simulink subsystem "MFTiresMultibodySSC"  (R2024b)
settings: Solver=VariableStepAuto  StartTime=0.0  StopTime=10.0  RelTol=1e-3
undefined symbols (not defined in the file): AxlFL, AxlFR, AxlRL, AxlRR, PlntVehMultiBody, WheelFL, WheelFR, WheelRL, WheelRR, X, Y, Z
libraries: sm_lib x68, nesl_utility x52, fl_lib x8
(part 3 of 3)

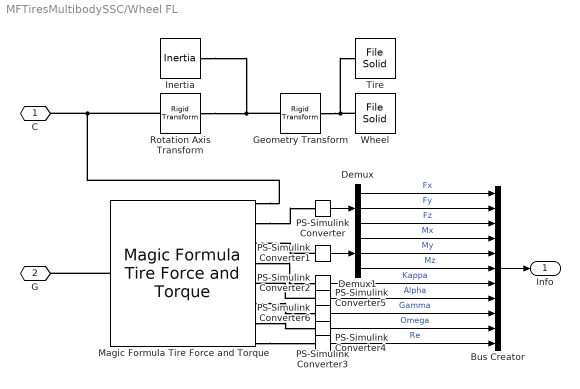
== system MFTiresMultibodySSC/Wheel FL ==
  Bus Creator : BusCreator  Inputs=11
  Demux : Demux  Outputs=3
  Demux1 : Demux  Outputs=3
  Geometry Transform : sm_lib/Frames and Transforms/Rigid Transform  RotationMethod=StandardAxis  FollAlignAxisA=+X  BaseAlignAxisA=+Y  FollAlignAxisB=+Y  BaseAlignAxisB=+Z  RotationStandardAxis=+X  RotationAngle=sideSign*180-90  RotationAngleUnits=deg  RotationArbitraryAxis=[0 0 1]  RotationSequenceAxes=FollowerAxes  RotationSequence=XYX  RotationSequenceAngles=[0 0 0]  RotationSequenceAnglesUnits=deg  RotationMatrix=[1 0 0; 0 1 0; 0 0 1]  Quaternion=[1 0 0 0]  TranslationMethod=StandardAxis  TranslationCartesianOffset=[0 0 0]  TranslationCartesianOffsetUnits=m  TranslationStandardAxis=+Y  TranslationStandardOffset=(1-2*sideSign)*0.125  TranslationStandardOffsetUnits=m  TranslationROffset=0  TranslationROffsetUnits=m  TranslationThetaOffset=0  TranslationThetaOffsetUnits=deg  TranslationZOffset=0  TranslationZOffsetUnits=m
  Inertia : sm_lib/Body Elements/Inertia  InertiaType=Custom  Mass=wheelAssm_mass  MassUnits=kg  CenterOfMass=[0 0 0]  CenterOfMassUnits=m  MomentsOfInertia=wheelAssm_I  MomentsOfInertiaUnits=kg*m^2  ProductsOfInertia=[0 0 0]  ProductsOfInertiaUnits=kg*m^2  GraphicType=None  MarkerShape=Inertia  MarkerSize=20  GraphicVisPropType=SimpleVisualProperties  GraphicDiffuseColor=[0.5 0.5 0.5]  GraphicOpacity=1.0  GraphicSpecularColor=[0.5 0.5 0.5 1.0]  GraphicAmbientColor=[0.15 0.15 0.15 1.0]  GraphicEmissiveColor=[0.0 0.0 0.0 1.0]  GraphicShininess=75
  Magic Formula Tire Force and Torque : sm_lib/Forces and Torques/Magic Formula Tire Force and Torque  TireSide=Left  TireParameters=tire_param  SlipMode=Combined  ContactFrameMethod=ClosestPoint  ScalingCoefficientLMUXMode=FromTireParameters  ScalingCoefficientLMUYMode=FromTireParameters  SenseContactSignal=off  TireWrenchFrame=ContactFrame  SenseTireForce=on  SenseTireTorque=on  SensePneumaticTrail=off  SenseLongitudinalSlip=on  SenseSaturatedLongitudinalSlip=off  SenseSlipAngle=on  SenseSaturatedSlipAngle=off  SenseTurnSlip=off  SenseRelativeLongitudinalVelocity=off  SenseRelativeLateralVelocity=off  SenseLongitudinalSlipVelocity=off  SenseLateralSlipVelocity=off  SenseYawVelocity=off  SenseCamberAngle=on  SenseSaturatedCamberAngle=off  SenseCamberVelocity=off  SenseSpinVelocity=on  SenseFreeRadius=off  SenseLoadedRadius=off  SenseEffectiveRollingRadius=on  SenseRadialDeflection=off  SenseLongitudinalFrictionCoefficient=off  SenseLateralFrictionCoefficient=off  SenseContactBaseRotation=off  SenseContactBaseTranslation=off  SenseContactFollowerRotation=off  SenseContactFollowerTranslation=off  NumericParameters=[0.1 0.1 0.1 0.1 0.1 1e-4 1e-4 1e-7 1e-7 1e-4 1e-4 0.1 1e-4 1e-4 1e-4 1e-4 1e-4 1e-4 1e-4 1e-4 1e-4]
  PS-Simulink Converter{,1..6} (7 alike) : nesl_utility/PS-Simulink Converter  PhysicalDomain=network_engine_domain  SubClassName=ps_output  LeftPortType=input  RightPortType=output  PseudoPeriodic=off  Frequencies=[]  VectorFormat=1-D array  Unit=inherit  AffineConversion=off
  Rotation Axis Transform : sm_lib/Frames and Transforms/Rigid Transform  RotationMethod=AlignedAxes  FollAlignAxisA=+X  BaseAlignAxisA=+X  FollAlignAxisB=+Z  BaseAlignAxisB=+Y  RotationStandardAxis=-X  RotationAngle=0  RotationAngleUnits=deg  RotationArbitraryAxis=[0 0 1]  RotationSequenceAxes=FollowerAxes  RotationSequence=XYX  RotationSequenceAngles=[0 0 0]  RotationSequenceAnglesUnits=deg  RotationMatrix=[1 0 0; 0 1 0; 0 0 1]  Quaternion=[1 0 0 0]  TranslationMethod=None  TranslationCartesianOffset=[0 0 0]  TranslationCartesianOffsetUnits=m  TranslationStandardAxis=+Z  TranslationStandardOffset=0  TranslationStandardOffsetUnits=m  TranslationROffset=0  TranslationROffsetUnits=m  TranslationThetaOffset=0  TranslationThetaOffsetUnits=deg  TranslationZOffset=0  TranslationZOffsetUnits=m
  Tire : sm_lib/Body Elements/File Solid  ExtGeomFileName=sm_car_heave_roll_tire.STL  UnitType=Custom  ExtGeomFileUnits=mm  StepReaderType=HEX  ExportConvexHullGeometry=off  InertiaType=Custom  BasedOnType=Density  Density=1000  DensityUnits=kg/m^3  Mass=0  MassUnits=kg  CenterOfMass=[0 0 0]  CenterOfMassUnits=m  MomentsOfInertia=[0 0 0]  MomentsOfInertiaUnits=kg*m^2  ProductsOfInertia=[0 0 0]  ProductsOfInertiaUnits=kg*m^2  GraphicType=FromGeometry  MarkerShape=Sphere  MarkerSize=10  GraphicVisPropType=SimpleVisualProperties  GraphicDiffuseColor=[0.5 0.5 0.5]  GraphicOpacity=1.0  GraphicSpecularColor=[0.5 0.5 0.5 1.0]  GraphicAmbientColor=[0.15 0.15 0.15 1.0]  GraphicEmissiveColor=[0.0 0.0 0.0 1.0]  GraphicShininess=75  DoExposeReferenceFrame=on  SerializedFrames=<Frames/>
  Wheel : sm_lib/Body Elements/File Solid  ExtGeomFileName=sm_car_heave_roll_wheel.STL  UnitType=Custom  ExtGeomFileUnits=mm  StepReaderType=HEX  ExportConvexHullGeometry=off  InertiaType=Custom  BasedOnType=Density  Density=1000  DensityUnits=kg/m^3  Mass=0  MassUnits=kg  CenterOfMass=[0 0 0]  CenterOfMassUnits=m  MomentsOfInertia=[0 0 0]  MomentsOfInertiaUnits=kg*m^2  ProductsOfInertia=[0 0 0]  ProductsOfInertiaUnits=kg*m^2  GraphicType=FromGeometry  MarkerShape=Sphere  MarkerSize=10  GraphicVisPropType=SimpleVisualProperties  GraphicDiffuseColor=[0.8 0.8 0.8]  GraphicOpacity=1.0  GraphicSpecularColor=[0.5 0.5 0.5 1.0]  GraphicAmbientColor=[0.15 0.15 0.15 1.0]  GraphicEmissiveColor=[0.0 0.0 0.0 1.0]  GraphicShininess=75  DoExposeReferenceFrame=on  SerializedFrames=<Frames/>
  C : PMIOPort  Side=Left
  G : PMIOPort  Port=2  Side=Right
  Info : Outport
  wires:
  PS-Simulink Converter5/1 -> Bus Creator/8  "Alpha"
  PS-Simulink Converter4/1 -> Bus Creator/11  "Re"
  PS-Simulink Converter3/1 -> Bus Creator/10  "Omega"
  PS-Simulink Converter2/1 -> Bus Creator/7  "Kappa"
  PS-Simulink Converter/1 -> Demux/1
  Demux/1 -> Bus Creator/1  "Fx"
  Demux/2 -> Bus Creator/2  "Fy"
  Demux/3 -> Bus Creator/3  "Fz"
  Demux1/3 -> Bus Creator/6  "Mz"
  Demux1/2 -> Bus Creator/5  "My"
  Demux1/1 -> Bus Creator/4  "Mx"
  PS-Simulink Converter1/1 -> Demux1/1
  Bus Creator/1 -> Info/1
  PS-Simulink Converter6/1 -> Bus Creator/9  "Gamma"
  connections:
  PS-Simulink Converter5/LConn1 -- Magic Formula Tire Force and Torque/RConn5
  Magic Formula Tire Force and Torque/RConn7 -- PS-Simulink Converter3/LConn1
  Magic Formula Tire Force and Torque/RConn8 -- PS-Simulink Converter4/LConn1
  Magic Formula Tire Force and Torque/RConn4 -- PS-Simulink Converter2/LConn1
  Wheel/RConn1 -- Geometry Transform/RConn1 -- Tire/RConn1
  Inertia/RConn1 -- Geometry Transform/LConn1 -- Rotation Axis Transform/LConn1
  Magic Formula Tire Force and Torque/LConn1 -- G/RConn1
  Magic Formula Tire Force and Torque/RConn2 -- PS-Simulink Converter/LConn1
  PS-Simulink Converter1/LConn1 -- Magic Formula Tire Force and Torque/RConn3
  Rotation Axis Transform/RConn1 -- Magic Formula Tire Force and Torque/RConn1 -- C/RConn1
  Magic Formula Tire Force and Torque/RConn6 -- PS-Simulink Converter6/LConn1

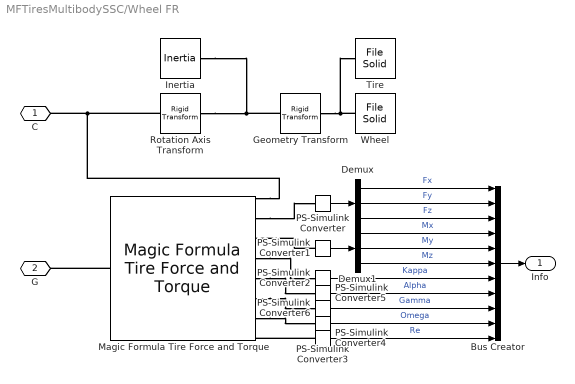
== system MFTiresMultibodySSC/Wheel FR ==
  Bus Creator : BusCreator  Inputs=11
  Demux : Demux  Outputs=3
  Demux1 : Demux  Outputs=3
  Geometry Transform : sm_lib/Frames and Transforms/Rigid Transform  RotationMethod=StandardAxis  FollAlignAxisA=+X  BaseAlignAxisA=+Y  FollAlignAxisB=+Y  BaseAlignAxisB=+Z  RotationStandardAxis=+X  RotationAngle=sideSign*180-90  RotationAngleUnits=deg  RotationArbitraryAxis=[0 0 1]  RotationSequenceAxes=FollowerAxes  RotationSequence=XYX  RotationSequenceAngles=[0 0 0]  RotationSequenceAnglesUnits=deg  RotationMatrix=[1 0 0; 0 1 0; 0 0 1]  Quaternion=[1 0 0 0]  TranslationMethod=StandardAxis  TranslationCartesianOffset=[0 0 0]  TranslationCartesianOffsetUnits=m  TranslationStandardAxis=+Y  TranslationStandardOffset=(1-2*sideSign)*0.125  TranslationStandardOffsetUnits=m  TranslationROffset=0  TranslationROffsetUnits=m  TranslationThetaOffset=0  TranslationThetaOffsetUnits=deg  TranslationZOffset=0  TranslationZOffsetUnits=m
  Inertia : sm_lib/Body Elements/Inertia  InertiaType=Custom  Mass=wheelAssm_mass  MassUnits=kg  CenterOfMass=[0 0 0]  CenterOfMassUnits=m  MomentsOfInertia=wheelAssm_I  MomentsOfInertiaUnits=kg*m^2  ProductsOfInertia=[0 0 0]  ProductsOfInertiaUnits=kg*m^2  GraphicType=None  MarkerShape=Inertia  MarkerSize=20  GraphicVisPropType=SimpleVisualProperties  GraphicDiffuseColor=[0.5 0.5 0.5]  GraphicOpacity=1.0  GraphicSpecularColor=[0.5 0.5 0.5 1.0]  GraphicAmbientColor=[0.15 0.15 0.15 1.0]  GraphicEmissiveColor=[0.0 0.0 0.0 1.0]  GraphicShininess=75
  Magic Formula Tire Force and Torque : sm_lib/Forces and Torques/Magic Formula Tire Force and Torque  TireSide=Right  TireParameters=tire_param  SlipMode=Combined  ContactFrameMethod=ClosestPoint  ScalingCoefficientLMUXMode=FromTireParameters  ScalingCoefficientLMUYMode=FromTireParameters  SenseContactSignal=off  TireWrenchFrame=ContactFrame  SenseTireForce=on  SenseTireTorque=on  SensePneumaticTrail=off  SenseLongitudinalSlip=on  SenseSaturatedLongitudinalSlip=off  SenseSlipAngle=on  SenseSaturatedSlipAngle=off  SenseTurnSlip=off  SenseRelativeLongitudinalVelocity=off  SenseRelativeLateralVelocity=off  SenseLongitudinalSlipVelocity=off  SenseLateralSlipVelocity=off  SenseYawVelocity=off  SenseCamberAngle=on  SenseSaturatedCamberAngle=off  SenseCamberVelocity=off  SenseSpinVelocity=on  SenseFreeRadius=off  SenseLoadedRadius=off  SenseEffectiveRollingRadius=on  SenseRadialDeflection=off  SenseLongitudinalFrictionCoefficient=off  SenseLateralFrictionCoefficient=off  SenseContactBaseRotation=off  SenseContactBaseTranslation=off  SenseContactFollowerRotation=off  SenseContactFollowerTranslation=off  NumericParameters=[0.1 0.1 0.1 0.1 0.1 1e-4 1e-4 1e-7 1e-7 1e-4 1e-4 0.1 1e-4 1e-4 1e-4 1e-4 1e-4 1e-4 1e-4 1e-4 1e-4]
  PS-Simulink Converter{,1..6} (7 alike) : nesl_utility/PS-Simulink Converter  PhysicalDomain=network_engine_domain  SubClassName=ps_output  LeftPortType=input  RightPortType=output  PseudoPeriodic=off  Frequencies=[]  VectorFormat=1-D array  Unit=inherit  AffineConversion=off
  Rotation Axis Transform : sm_lib/Frames and Transforms/Rigid Transform  RotationMethod=AlignedAxes  FollAlignAxisA=+X  BaseAlignAxisA=+X  FollAlignAxisB=+Z  BaseAlignAxisB=+Y  RotationStandardAxis=-X  RotationAngle=0  RotationAngleUnits=deg  RotationArbitraryAxis=[0 0 1]  RotationSequenceAxes=FollowerAxes  RotationSequence=XYX  RotationSequenceAngles=[0 0 0]  RotationSequenceAnglesUnits=deg  RotationMatrix=[1 0 0; 0 1 0; 0 0 1]  Quaternion=[1 0 0 0]  TranslationMethod=None  TranslationCartesianOffset=[0 0 0]  TranslationCartesianOffsetUnits=m  TranslationStandardAxis=+Z  TranslationStandardOffset=0  TranslationStandardOffsetUnits=m  TranslationROffset=0  TranslationROffsetUnits=m  TranslationThetaOffset=0  TranslationThetaOffsetUnits=deg  TranslationZOffset=0  TranslationZOffsetUnits=m
  Tire : sm_lib/Body Elements/File Solid  ExtGeomFileName=sm_car_heave_roll_tire.STL  UnitType=Custom  ExtGeomFileUnits=mm  StepReaderType=HEX  ExportConvexHullGeometry=off  InertiaType=Custom  BasedOnType=Density  Density=1000  DensityUnits=kg/m^3  Mass=0  MassUnits=kg  CenterOfMass=[0 0 0]  CenterOfMassUnits=m  MomentsOfInertia=[0 0 0]  MomentsOfInertiaUnits=kg*m^2  ProductsOfInertia=[0 0 0]  ProductsOfInertiaUnits=kg*m^2  GraphicType=FromGeometry  MarkerShape=Sphere  MarkerSize=10  GraphicVisPropType=SimpleVisualProperties  GraphicDiffuseColor=[0.5 0.5 0.5]  GraphicOpacity=1.0  GraphicSpecularColor=[0.5 0.5 0.5 1.0]  GraphicAmbientColor=[0.15 0.15 0.15 1.0]  GraphicEmissiveColor=[0.0 0.0 0.0 1.0]  GraphicShininess=75  DoExposeReferenceFrame=on  SerializedFrames=<Frames/>
  Wheel : sm_lib/Body Elements/File Solid  ExtGeomFileName=sm_car_heave_roll_wheel.STL  UnitType=Custom  ExtGeomFileUnits=mm  StepReaderType=HEX  ExportConvexHullGeometry=off  InertiaType=Custom  BasedOnType=Density  Density=1000  DensityUnits=kg/m^3  Mass=0  MassUnits=kg  CenterOfMass=[0 0 0]  CenterOfMassUnits=m  MomentsOfInertia=[0 0 0]  MomentsOfInertiaUnits=kg*m^2  ProductsOfInertia=[0 0 0]  ProductsOfInertiaUnits=kg*m^2  GraphicType=FromGeometry  MarkerShape=Sphere  MarkerSize=10  GraphicVisPropType=SimpleVisualProperties  GraphicDiffuseColor=[0.8 0.8 0.8]  GraphicOpacity=1.0  GraphicSpecularColor=[0.5 0.5 0.5 1.0]  GraphicAmbientColor=[0.15 0.15 0.15 1.0]  GraphicEmissiveColor=[0.0 0.0 0.0 1.0]  GraphicShininess=75  DoExposeReferenceFrame=on  SerializedFrames=<Frames/>
  C : PMIOPort  Side=Left
  G : PMIOPort  Port=2  Side=Right
  Info : Outport
  wires:
  PS-Simulink Converter5/1 -> Bus Creator/8  "Alpha"
  PS-Simulink Converter4/1 -> Bus Creator/11  "Re"
  PS-Simulink Converter3/1 -> Bus Creator/10  "Omega"
  PS-Simulink Converter2/1 -> Bus Creator/7  "Kappa"
  PS-Simulink Converter/1 -> Demux/1
  Demux/1 -> Bus Creator/1  "Fx"
  Demux/2 -> Bus Creator/2  "Fy"
  Demux/3 -> Bus Creator/3  "Fz"
  Demux1/3 -> Bus Creator/6  "Mz"
  Demux1/2 -> Bus Creator/5  "My"
  Demux1/1 -> Bus Creator/4  "Mx"
  PS-Simulink Converter1/1 -> Demux1/1
  Bus Creator/1 -> Info/1
  PS-Simulink Converter6/1 -> Bus Creator/9  "Gamma"
  connections:
  Magic Formula Tire Force and Torque/RConn5 -- PS-Simulink Converter5/LConn1
  PS-Simulink Converter4/LConn1 -- Magic Formula Tire Force and Torque/RConn8
  Magic Formula Tire Force and Torque/RConn7 -- PS-Simulink Converter3/LConn1
  Magic Formula Tire Force and Torque/RConn4 -- PS-Simulink Converter2/LConn1
  Wheel/RConn1 -- Geometry Transform/RConn1 -- Tire/RConn1
  Inertia/RConn1 -- Geometry Transform/LConn1 -- Rotation Axis Transform/LConn1
  Magic Formula Tire Force and Torque/LConn1 -- G/RConn1
  Magic Formula Tire Force and Torque/RConn2 -- PS-Simulink Converter/LConn1
  PS-Simulink Converter1/LConn1 -- Magic Formula Tire Force and Torque/RConn3
  Rotation Axis Transform/RConn1 -- Magic Formula Tire Force and Torque/RConn1 -- C/RConn1
  Magic Formula Tire Force and Torque/RConn6 -- PS-Simulink Converter6/LConn1

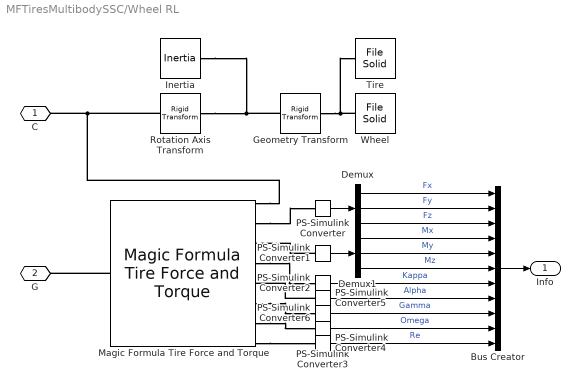
== system MFTiresMultibodySSC/Wheel RL ==
  Bus Creator : BusCreator  Inputs=11
  Demux : Demux  Outputs=3
  Demux1 : Demux  Outputs=3
  Geometry Transform : sm_lib/Frames and Transforms/Rigid Transform  RotationMethod=StandardAxis  FollAlignAxisA=+X  BaseAlignAxisA=+Y  FollAlignAxisB=+Y  BaseAlignAxisB=+Z  RotationStandardAxis=+X  RotationAngle=sideSign*180-90  RotationAngleUnits=deg  RotationArbitraryAxis=[0 0 1]  RotationSequenceAxes=FollowerAxes  RotationSequence=XYX  RotationSequenceAngles=[0 0 0]  RotationSequenceAnglesUnits=deg  RotationMatrix=[1 0 0; 0 1 0; 0 0 1]  Quaternion=[1 0 0 0]  TranslationMethod=StandardAxis  TranslationCartesianOffset=[0 0 0]  TranslationCartesianOffsetUnits=m  TranslationStandardAxis=+Y  TranslationStandardOffset=(1-2*sideSign)*0.125  TranslationStandardOffsetUnits=m  TranslationROffset=0  TranslationROffsetUnits=m  TranslationThetaOffset=0  TranslationThetaOffsetUnits=deg  TranslationZOffset=0  TranslationZOffsetUnits=m
  Inertia : sm_lib/Body Elements/Inertia  InertiaType=Custom  Mass=wheelAssm_mass  MassUnits=kg  CenterOfMass=[0 0 0]  CenterOfMassUnits=m  MomentsOfInertia=wheelAssm_I  MomentsOfInertiaUnits=kg*m^2  ProductsOfInertia=[0 0 0]  ProductsOfInertiaUnits=kg*m^2  GraphicType=None  MarkerShape=Inertia  MarkerSize=20  GraphicVisPropType=SimpleVisualProperties  GraphicDiffuseColor=[0.5 0.5 0.5]  GraphicOpacity=1.0  GraphicSpecularColor=[0.5 0.5 0.5 1.0]  GraphicAmbientColor=[0.15 0.15 0.15 1.0]  GraphicEmissiveColor=[0.0 0.0 0.0 1.0]  GraphicShininess=75
  Magic Formula Tire Force and Torque : sm_lib/Forces and Torques/Magic Formula Tire Force and Torque  TireSide=Left  TireParameters=tire_param  SlipMode=Combined  ContactFrameMethod=ClosestPoint  ScalingCoefficientLMUXMode=FromTireParameters  ScalingCoefficientLMUYMode=FromTireParameters  SenseContactSignal=off  TireWrenchFrame=ContactFrame  SenseTireForce=on  SenseTireTorque=on  SensePneumaticTrail=off  SenseLongitudinalSlip=on  SenseSaturatedLongitudinalSlip=off  SenseSlipAngle=on  SenseSaturatedSlipAngle=off  SenseTurnSlip=off  SenseRelativeLongitudinalVelocity=off  SenseRelativeLateralVelocity=off  SenseLongitudinalSlipVelocity=off  SenseLateralSlipVelocity=off  SenseYawVelocity=off  SenseCamberAngle=on  SenseSaturatedCamberAngle=off  SenseCamberVelocity=off  SenseSpinVelocity=on  SenseFreeRadius=off  SenseLoadedRadius=off  SenseEffectiveRollingRadius=on  SenseRadialDeflection=off  SenseLongitudinalFrictionCoefficient=off  SenseLateralFrictionCoefficient=off  SenseContactBaseRotation=off  SenseContactBaseTranslation=off  SenseContactFollowerRotation=off  SenseContactFollowerTranslation=off  NumericParameters=[0.1 0.1 0.1 0.1 0.1 1e-4 1e-4 1e-7 1e-7 1e-4 1e-4 0.1 1e-4 1e-4 1e-4 1e-4 1e-4 1e-4 1e-4 1e-4 1e-4]
  PS-Simulink Converter{,1..6} (7 alike) : nesl_utility/PS-Simulink Converter  PhysicalDomain=network_engine_domain  SubClassName=ps_output  LeftPortType=input  RightPortType=output  PseudoPeriodic=off  Frequencies=[]  VectorFormat=1-D array  Unit=inherit  AffineConversion=off
  Rotation Axis Transform : sm_lib/Frames and Transforms/Rigid Transform  RotationMethod=AlignedAxes  FollAlignAxisA=+X  BaseAlignAxisA=+X  FollAlignAxisB=+Z  BaseAlignAxisB=+Y  RotationStandardAxis=-X  RotationAngle=0  RotationAngleUnits=deg  RotationArbitraryAxis=[0 0 1]  RotationSequenceAxes=FollowerAxes  RotationSequence=XYX  RotationSequenceAngles=[0 0 0]  RotationSequenceAnglesUnits=deg  RotationMatrix=[1 0 0; 0 1 0; 0 0 1]  Quaternion=[1 0 0 0]  TranslationMethod=None  TranslationCartesianOffset=[0 0 0]  TranslationCartesianOffsetUnits=m  TranslationStandardAxis=+Z  TranslationStandardOffset=0  TranslationStandardOffsetUnits=m  TranslationROffset=0  TranslationROffsetUnits=m  TranslationThetaOffset=0  TranslationThetaOffsetUnits=deg  TranslationZOffset=0  TranslationZOffsetUnits=m
  Tire : sm_lib/Body Elements/File Solid  ExtGeomFileName=sm_car_heave_roll_tire.STL  UnitType=Custom  ExtGeomFileUnits=mm  StepReaderType=HEX  ExportConvexHullGeometry=off  InertiaType=Custom  BasedOnType=Density  Density=1000  DensityUnits=kg/m^3  Mass=0  MassUnits=kg  CenterOfMass=[0 0 0]  CenterOfMassUnits=m  MomentsOfInertia=[0 0 0]  MomentsOfInertiaUnits=kg*m^2  ProductsOfInertia=[0 0 0]  ProductsOfInertiaUnits=kg*m^2  GraphicType=FromGeometry  MarkerShape=Sphere  MarkerSize=10  GraphicVisPropType=SimpleVisualProperties  GraphicDiffuseColor=[0.5 0.5 0.5]  GraphicOpacity=1.0  GraphicSpecularColor=[0.5 0.5 0.5 1.0]  GraphicAmbientColor=[0.15 0.15 0.15 1.0]  GraphicEmissiveColor=[0.0 0.0 0.0 1.0]  GraphicShininess=75  DoExposeReferenceFrame=on  SerializedFrames=<Frames/>
  Wheel : sm_lib/Body Elements/File Solid  ExtGeomFileName=sm_car_heave_roll_wheel.STL  UnitType=Custom  ExtGeomFileUnits=mm  StepReaderType=HEX  ExportConvexHullGeometry=off  InertiaType=Custom  BasedOnType=Density  Density=1000  DensityUnits=kg/m^3  Mass=0  MassUnits=kg  CenterOfMass=[0 0 0]  CenterOfMassUnits=m  MomentsOfInertia=[0 0 0]  MomentsOfInertiaUnits=kg*m^2  ProductsOfInertia=[0 0 0]  ProductsOfInertiaUnits=kg*m^2  GraphicType=FromGeometry  MarkerShape=Sphere  MarkerSize=10  GraphicVisPropType=SimpleVisualProperties  GraphicDiffuseColor=[0.8 0.8 0.8]  GraphicOpacity=1.0  GraphicSpecularColor=[0.5 0.5 0.5 1.0]  GraphicAmbientColor=[0.15 0.15 0.15 1.0]  GraphicEmissiveColor=[0.0 0.0 0.0 1.0]  GraphicShininess=75  DoExposeReferenceFrame=on  SerializedFrames=<Frames/>
  C : PMIOPort  Side=Left
  G : PMIOPort  Port=2  Side=Right
  Info : Outport
  wires:
  PS-Simulink Converter5/1 -> Bus Creator/8  "Alpha"
  PS-Simulink Converter4/1 -> Bus Creator/11  "Re"
  PS-Simulink Converter3/1 -> Bus Creator/10  "Omega"
  PS-Simulink Converter2/1 -> Bus Creator/7  "Kappa"
  PS-Simulink Converter/1 -> Demux/1
  Demux/1 -> Bus Creator/1  "Fx"
  Demux/2 -> Bus Creator/2  "Fy"
  Demux/3 -> Bus Creator/3  "Fz"
  Demux1/3 -> Bus Creator/6  "Mz"
  Demux1/2 -> Bus Creator/5  "My"
  Demux1/1 -> Bus Creator/4  "Mx"
  PS-Simulink Converter1/1 -> Demux1/1
  Bus Creator/1 -> Info/1
  PS-Simulink Converter6/1 -> Bus Creator/9  "Gamma"
  connections:
  PS-Simulink Converter5/LConn1 -- Magic Formula Tire Force and Torque/RConn5
  Magic Formula Tire Force and Torque/RConn7 -- PS-Simulink Converter3/LConn1
  Magic Formula Tire Force and Torque/RConn8 -- PS-Simulink Converter4/LConn1
  Magic Formula Tire Force and Torque/RConn4 -- PS-Simulink Converter2/LConn1
  Wheel/RConn1 -- Geometry Transform/RConn1 -- Tire/RConn1
  Inertia/RConn1 -- Geometry Transform/LConn1 -- Rotation Axis Transform/LConn1
  Magic Formula Tire Force and Torque/LConn1 -- G/RConn1
  Magic Formula Tire Force and Torque/RConn2 -- PS-Simulink Converter/LConn1
  PS-Simulink Converter1/LConn1 -- Magic Formula Tire Force and Torque/RConn3
  Rotation Axis Transform/RConn1 -- Magic Formula Tire Force and Torque/RConn1 -- C/RConn1
  Magic Formula Tire Force and Torque/RConn6 -- PS-Simulink Converter6/LConn1

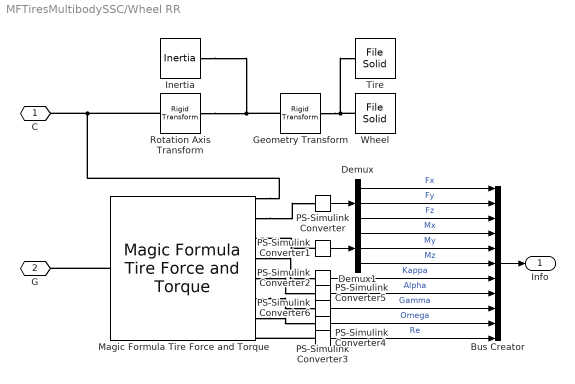
== system MFTiresMultibodySSC/Wheel RR ==
  Bus Creator : BusCreator  Inputs=11
  Demux : Demux  Outputs=3
  Demux1 : Demux  Outputs=3
  Geometry Transform : sm_lib/Frames and Transforms/Rigid Transform  RotationMethod=StandardAxis  FollAlignAxisA=+X  BaseAlignAxisA=+Y  FollAlignAxisB=+Y  BaseAlignAxisB=+Z  RotationStandardAxis=+X  RotationAngle=sideSign*180-90  RotationAngleUnits=deg  RotationArbitraryAxis=[0 0 1]  RotationSequenceAxes=FollowerAxes  RotationSequence=XYX  RotationSequenceAngles=[0 0 0]  RotationSequenceAnglesUnits=deg  RotationMatrix=[1 0 0; 0 1 0; 0 0 1]  Quaternion=[1 0 0 0]  TranslationMethod=StandardAxis  TranslationCartesianOffset=[0 0 0]  TranslationCartesianOffsetUnits=m  TranslationStandardAxis=+Y  TranslationStandardOffset=(1-2*sideSign)*0.125  TranslationStandardOffsetUnits=m  TranslationROffset=0  TranslationROffsetUnits=m  TranslationThetaOffset=0  TranslationThetaOffsetUnits=deg  TranslationZOffset=0  TranslationZOffsetUnits=m
  Inertia : sm_lib/Body Elements/Inertia  InertiaType=Custom  Mass=wheelAssm_mass  MassUnits=kg  CenterOfMass=[0 0 0]  CenterOfMassUnits=m  MomentsOfInertia=wheelAssm_I  MomentsOfInertiaUnits=kg*m^2  ProductsOfInertia=[0 0 0]  ProductsOfInertiaUnits=kg*m^2  GraphicType=None  MarkerShape=Inertia  MarkerSize=20  GraphicVisPropType=SimpleVisualProperties  GraphicDiffuseColor=[0.5 0.5 0.5]  GraphicOpacity=1.0  GraphicSpecularColor=[0.5 0.5 0.5 1.0]  GraphicAmbientColor=[0.15 0.15 0.15 1.0]  GraphicEmissiveColor=[0.0 0.0 0.0 1.0]  GraphicShininess=75
  Magic Formula Tire Force and Torque : sm_lib/Forces and Torques/Magic Formula Tire Force and Torque  TireSide=Right  TireParameters=tire_param  SlipMode=Combined  ContactFrameMethod=ClosestPoint  ScalingCoefficientLMUXMode=FromTireParameters  ScalingCoefficientLMUYMode=FromTireParameters  SenseContactSignal=off  TireWrenchFrame=ContactFrame  SenseTireForce=on  SenseTireTorque=on  SensePneumaticTrail=off  SenseLongitudinalSlip=on  SenseSaturatedLongitudinalSlip=off  SenseSlipAngle=on  SenseSaturatedSlipAngle=off  SenseTurnSlip=off  SenseRelativeLongitudinalVelocity=off  SenseRelativeLateralVelocity=off  SenseLongitudinalSlipVelocity=off  SenseLateralSlipVelocity=off  SenseYawVelocity=off  SenseCamberAngle=on  SenseSaturatedCamberAngle=off  SenseCamberVelocity=off  SenseSpinVelocity=on  SenseFreeRadius=off  SenseLoadedRadius=off  SenseEffectiveRollingRadius=on  SenseRadialDeflection=off  SenseLongitudinalFrictionCoefficient=off  SenseLateralFrictionCoefficient=off  SenseContactBaseRotation=off  SenseContactBaseTranslation=off  SenseContactFollowerRotation=off  SenseContactFollowerTranslation=off  NumericParameters=[0.1 0.1 0.1 0.1 0.1 1e-4 1e-4 1e-7 1e-7 1e-4 1e-4 0.1 1e-4 1e-4 1e-4 1e-4 1e-4 1e-4 1e-4 1e-4 1e-4]
  PS-Simulink Converter{,1..6} (7 alike) : nesl_utility/PS-Simulink Converter  PhysicalDomain=network_engine_domain  SubClassName=ps_output  LeftPortType=input  RightPortType=output  PseudoPeriodic=off  Frequencies=[]  VectorFormat=1-D array  Unit=inherit  AffineConversion=off
  Rotation Axis Transform : sm_lib/Frames and Transforms/Rigid Transform  RotationMethod=AlignedAxes  FollAlignAxisA=+X  BaseAlignAxisA=+X  FollAlignAxisB=+Z  BaseAlignAxisB=+Y  RotationStandardAxis=-X  RotationAngle=0  RotationAngleUnits=deg  RotationArbitraryAxis=[0 0 1]  RotationSequenceAxes=FollowerAxes  RotationSequence=XYX  RotationSequenceAngles=[0 0 0]  RotationSequenceAnglesUnits=deg  RotationMatrix=[1 0 0; 0 1 0; 0 0 1]  Quaternion=[1 0 0 0]  TranslationMethod=None  TranslationCartesianOffset=[0 0 0]  TranslationCartesianOffsetUnits=m  TranslationStandardAxis=+Z  TranslationStandardOffset=0  TranslationStandardOffsetUnits=m  TranslationROffset=0  TranslationROffsetUnits=m  TranslationThetaOffset=0  TranslationThetaOffsetUnits=deg  TranslationZOffset=0  TranslationZOffsetUnits=m
  Tire : sm_lib/Body Elements/File Solid  ExtGeomFileName=sm_car_heave_roll_tire.STL  UnitType=Custom  ExtGeomFileUnits=mm  StepReaderType=HEX  ExportConvexHullGeometry=off  InertiaType=Custom  BasedOnType=Density  Density=1000  DensityUnits=kg/m^3  Mass=0  MassUnits=kg  CenterOfMass=[0 0 0]  CenterOfMassUnits=m  MomentsOfInertia=[0 0 0]  MomentsOfInertiaUnits=kg*m^2  ProductsOfInertia=[0 0 0]  ProductsOfInertiaUnits=kg*m^2  GraphicType=FromGeometry  MarkerShape=Sphere  MarkerSize=10  GraphicVisPropType=SimpleVisualProperties  GraphicDiffuseColor=[0.5 0.5 0.5]  GraphicOpacity=1.0  GraphicSpecularColor=[0.5 0.5 0.5 1.0]  GraphicAmbientColor=[0.15 0.15 0.15 1.0]  GraphicEmissiveColor=[0.0 0.0 0.0 1.0]  GraphicShininess=75  DoExposeReferenceFrame=on  SerializedFrames=<Frames/>
  Wheel : sm_lib/Body Elements/File Solid  ExtGeomFileName=sm_car_heave_roll_wheel.STL  UnitType=Custom  ExtGeomFileUnits=mm  StepReaderType=HEX  ExportConvexHullGeometry=off  InertiaType=Custom  BasedOnType=Density  Density=1000  DensityUnits=kg/m^3  Mass=0  MassUnits=kg  CenterOfMass=[0 0 0]  CenterOfMassUnits=m  MomentsOfInertia=[0 0 0]  MomentsOfInertiaUnits=kg*m^2  ProductsOfInertia=[0 0 0]  ProductsOfInertiaUnits=kg*m^2  GraphicType=FromGeometry  MarkerShape=Sphere  MarkerSize=10  GraphicVisPropType=SimpleVisualProperties  GraphicDiffuseColor=[0.8 0.8 0.8]  GraphicOpacity=1.0  GraphicSpecularColor=[0.5 0.5 0.5 1.0]  GraphicAmbientColor=[0.15 0.15 0.15 1.0]  GraphicEmissiveColor=[0.0 0.0 0.0 1.0]  GraphicShininess=75  DoExposeReferenceFrame=on  SerializedFrames=<Frames/>
  C : PMIOPort  Side=Left
  G : PMIOPort  Port=2  Side=Right
  Info : Outport
  wires:
  PS-Simulink Converter5/1 -> Bus Creator/8  "Alpha"
  PS-Simulink Converter4/1 -> Bus Creator/11  "Re"
  PS-Simulink Converter3/1 -> Bus Creator/10  "Omega"
  PS-Simulink Converter2/1 -> Bus Creator/7  "Kappa"
  PS-Simulink Converter/1 -> Demux/1
  Demux/1 -> Bus Creator/1  "Fx"
  Demux/2 -> Bus Creator/2  "Fy"
  Demux/3 -> Bus Creator/3  "Fz"
  Demux1/3 -> Bus Creator/6  "Mz"
  Demux1/2 -> Bus Creator/5  "My"
  Demux1/1 -> Bus Creator/4  "Mx"
  PS-Simulink Converter1/1 -> Demux1/1
  Bus Creator/1 -> Info/1
  PS-Simulink Converter6/1 -> Bus Creator/9  "Gamma"
  connections:
  Magic Formula Tire Force and Torque/RConn5 -- PS-Simulink Converter5/LConn1
  PS-Simulink Converter4/LConn1 -- Magic Formula Tire Force and Torque/RConn8
  Magic Formula Tire Force and Torque/RConn7 -- PS-Simulink Converter3/LConn1
  Magic Formula Tire Force and Torque/RConn4 -- PS-Simulink Converter2/LConn1
  Wheel/RConn1 -- Geometry Transform/RConn1 -- Tire/RConn1
  Inertia/RConn1 -- Geometry Transform/LConn1 -- Rotation Axis Transform/LConn1
  Magic Formula Tire Force and Torque/LConn1 -- G/RConn1
  Magic Formula Tire Force and Torque/RConn2 -- PS-Simulink Converter/LConn1
  PS-Simulink Converter1/LConn1 -- Magic Formula Tire Force and Torque/RConn3
  Rotation Axis Transform/RConn1 -- Magic Formula Tire Force and Torque/RConn1 -- C/RConn1
  Magic Formula Tire Force and Torque/RConn6 -- PS-Simulink Converter6/LConn1

== system MFTiresMultibodySSC/Bus Creation/Alpha ==
  Info : Inport
  Bus Selector : BusSelector  OutputSignals=FL.Alpha,FR.Alpha,RL.Alpha,RR.Alpha
  Vector Concatenate : Concatenate  NumInputs=4
  Alpha : Outport  VectorParamsAs1DForOutWhenUnconnected=off
  wires:
  Bus Selector/3 -> Vector Concatenate/3  "<Alpha>"
  Bus Selector/4 -> Vector Concatenate/4  "<Alpha>"
  Vector Concatenate/1 -> Alpha/1
  Info/1 -> Bus Selector/1
  Bus Selector/2 -> Vector Concatenate/2  "<Alpha>"
  Bus Selector/1 -> Vector Concatenate/1  "<Alpha>"

== system MFTiresMultibodySSC/Bus Creation/BrkPrs1 ==
  In1 : Inport
  BrkPrs : Outport  VectorParamsAs1DForOutWhenUnconnected=off
  wires:
  In1/1 -> BrkPrs/1  "BrkPrs"

== system MFTiresMultibodySSC/Bus Creation/Fx ==
  Info : Inport
  Bus Selector : BusSelector  OutputSignals=FL.Fx,FR.Fx,RL.Fx,RR.Fx
  Vector Concatenate : Concatenate  NumInputs=4
  Fx : Outport  VectorParamsAs1DForOutWhenUnconnected=off
  wires:
  Bus Selector/4 -> Vector Concatenate/4  "<Fx>"
  Bus Selector/3 -> Vector Concatenate/3  "<Fx>"
  Bus Selector/1 -> Vector Concatenate/1  "<Fx>"
  Info/1 -> Bus Selector/1
  Vector Concatenate/1 -> Fx/1
  Bus Selector/2 -> Vector Concatenate/2  "<Fx>"

== system MFTiresMultibodySSC/Bus Creation/Fy ==
  Info : Inport
  Bus Selector : BusSelector  OutputSignals=FL.Fy,FR.Fy,RL.Fy,RR.Fy
  Vector Concatenate : Concatenate  NumInputs=4
  Fy : Outport  VectorParamsAs1DForOutWhenUnconnected=off
  wires:
  Bus Selector/2 -> Vector Concatenate/2  "<Fy>"
  Bus Selector/4 -> Vector Concatenate/4  "<Fy>"
  Bus Selector/1 -> Vector Concatenate/1  "<Fy>"
  Bus Selector/3 -> Vector Concatenate/3  "<Fy>"
  Vector Concatenate/1 -> Fy/1
  Info/1 -> Bus Selector/1

== system MFTiresMultibodySSC/Bus Creation/Fz ==
  Info : Inport
  Bus Selector : BusSelector  OutputSignals=FL.Fz,FR.Fz,RL.Fz,RR.Fz
  Vector Concatenate : Concatenate  NumInputs=4
  Fz : Outport  VectorParamsAs1DForOutWhenUnconnected=off
  wires:
  Bus Selector/2 -> Vector Concatenate/2  "<Fz>"
  Bus Selector/4 -> Vector Concatenate/4  "<Fz>"
  Bus Selector/1 -> Vector Concatenate/1  "<Fz>"
  Bus Selector/3 -> Vector Concatenate/3  "<Fz>"
  Vector Concatenate/1 -> Fz/1
  Info/1 -> Bus Selector/1

== system MFTiresMultibodySSC/Bus Creation/Gamma ==
  Info : Inport
  Bus Selector : BusSelector  OutputSignals=FL.Gamma,FR.Gamma,RL.Gamma,RR.Gamma
  Vector Concatenate : Concatenate  NumInputs=4
  Gamma : Outport  VectorParamsAs1DForOutWhenUnconnected=off
  wires:
  Bus Selector/1 -> Vector Concatenate/1  "<Gamma>"
  Bus Selector/2 -> Vector Concatenate/2  "<Gamma>"
  Info/1 -> Bus Selector/1
  Vector Concatenate/1 -> Gamma/1
  Bus Selector/4 -> Vector Concatenate/4  "<Gamma>"
  Bus Selector/3 -> Vector Concatenate/3  "<Gamma>"

== system MFTiresMultibodySSC/Bus Creation/Kappa ==
  Info : Inport
  Bus Selector : BusSelector  OutputSignals=FL.Kappa,FR.Kappa,RL.Kappa,RR.Kappa
  Vector Concatenate : Concatenate  NumInputs=4
  Kappa : Outport  VectorParamsAs1DForOutWhenUnconnected=off
  wires:
  Bus Selector/3 -> Vector Concatenate/3  "<Kappa>"
  Bus Selector/4 -> Vector Concatenate/4  "<Kappa>"
  Vector Concatenate/1 -> Kappa/1
  Info/1 -> Bus Selector/1
  Bus Selector/2 -> Vector Concatenate/2  "<Kappa>"
  Bus Selector/1 -> Vector Concatenate/1  "<Kappa>"

== system MFTiresMultibodySSC/Bus Creation/Mx ==
  Info : Inport
  Bus Selector : BusSelector  OutputSignals=FL.Mx,FR.Mx,RL.Mx,RR.Mx
  Vector Concatenate : Concatenate  NumInputs=4
  Mx : Outport  VectorParamsAs1DForOutWhenUnconnected=off
  wires:
  Bus Selector/2 -> Vector Concatenate/2  "<Mx>"
  Bus Selector/4 -> Vector Concatenate/4  "<Mx>"
  Bus Selector/1 -> Vector Concatenate/1  "<Mx>"
  Bus Selector/3 -> Vector Concatenate/3  "<Mx>"
  Vector Concatenate/1 -> Mx/1
  Info/1 -> Bus Selector/1

== system MFTiresMultibodySSC/Bus Creation/My ==
  Info : Inport
  Bus Selector : BusSelector  OutputSignals=FL.My,FR.My,RL.My,RR.My
  Vector Concatenate : Concatenate  NumInputs=4
  My : Outport  VectorParamsAs1DForOutWhenUnconnected=off
  wires:
  Bus Selector/2 -> Vector Concatenate/2  "<My>"
  Bus Selector/4 -> Vector Concatenate/4  "<My>"
  Bus Selector/1 -> Vector Concatenate/1  "<My>"
  Bus Selector/3 -> Vector Concatenate/3  "<My>"
  Vector Concatenate/1 -> My/1
  Info/1 -> Bus Selector/1

== system MFTiresMultibodySSC/Bus Creation/Mz ==
  Info : Inport
  Bus Selector : BusSelector  OutputSignals=FL.Mz,FR.Mz,RL.Mz,RR.Mz
  Vector Concatenate : Concatenate  NumInputs=4
  Mz : Outport  VectorParamsAs1DForOutWhenUnconnected=off
  wires:
  Bus Selector/2 -> Vector Concatenate/2  "<Mz>"
  Bus Selector/4 -> Vector Concatenate/4  "<Mz>"
  Bus Selector/1 -> Vector Concatenate/1  "<Mz>"
  Bus Selector/3 -> Vector Concatenate/3  "<Mz>"
  Vector Concatenate/1 -> Mz/1
  Info/1 -> Bus Selector/1

== system MFTiresMultibodySSC/Bus Creation/Omega ==
  Info : Inport
  Bus Selector : BusSelector  OutputSignals=FL.Omega,FR.Omega,RL.Omega,RR.Omega
  Vector Concatenate : Concatenate  NumInputs=4
  Omega : Outport  VectorParamsAs1DForOutWhenUnconnected=off
  wires:
  Bus Selector/2 -> Vector Concatenate/2  "<Omega>"
  Bus Selector/4 -> Vector Concatenate/4  "<Omega>"
  Bus Selector/1 -> Vector Concatenate/1  "<Omega>"
  Bus Selector/3 -> Vector Concatenate/3  "<Omega>"
  Vector Concatenate/1 -> Omega/1
  Info/1 -> Bus Selector/1

== system MFTiresMultibodySSC/Bus Creation/Re ==
  Info : Inport
  Bus Selector : BusSelector  OutputSignals=FL.Re,FR.Re,RL.Re,RR.Re
  Vector Concatenate : Concatenate  NumInputs=4
  Re : Outport  VectorParamsAs1DForOutWhenUnconnected=off
  wires:
  Bus Selector/3 -> Vector Concatenate/3  "<Re>"
  Bus Selector/4 -> Vector Concatenate/4  "<Re>"
  Vector Concatenate/1 -> Re/1
  Info/1 -> Bus Selector/1
  Bus Selector/2 -> Vector Concatenate/2  "<Re>"
  Bus Selector/1 -> Vector Concatenate/1  "<Re>"

== system MFTiresMultibodySSC/Bus Creation/z ==
  Constant{,1..3} (4 alike) : Constant  Value=0  SampleTime=-1
  Vector Concatenate : Concatenate  NumInputs=4
  Out1 : Outport  VectorParamsAs1DForOutWhenUnconnected=off
  wires:
  Vector Concatenate/1 -> Out1/1
  Constant/1 -> Vector Concatenate/1  "z"
  Constant1/1 -> Vector Concatenate/2  "z"
  Constant2/1 -> Vector Concatenate/3  "z"
  Constant3/1 -> Vector Concatenate/4  "z"

== system MFTiresMultibodySSC/Bus Creation/zdot ==
  Constant{,1..3} (4 alike) : Constant  Value=0  SampleTime=-1
  Vector Concatenate : Concatenate  NumInputs=4
  Out1 : Outport  VectorParamsAs1DForOutWhenUnconnected=off
  wires:
  Constant3/1 -> Vector Concatenate/4  "zdot"
  Constant2/1 -> Vector Concatenate/3  "zdot"
  Constant1/1 -> Vector Concatenate/2  "zdot"
  Constant/1 -> Vector Concatenate/1  "zdot"
  Vector Concatenate/1 -> Out1/1
